simulink model "inversor"  (R2017a)
settings: Solver=FixedStepAuto  StartTime=0.0  StopTime=10.0  FixedStep=1/60/10000  RelTol=1e-3
undefined symbols (not defined in the file): C1, L1, La, R1
libraries: powerlib x15, powerlib_extras x1, simulink x1
settings Model: Creator=Administrador  LastModifiedBy=Administrador
settings OptimizationCC: DefaultParameterBehavior=Inlined  PassReuseOutputArgsAs=Individual arguments
settings DebuggingCC: ParameterTunabilityLossMsg=error
settings SFSimCC: MATLABDynamicMemAlloc=off
settings RTWCC: SystemTargetFile=ert.tlc  TemplateMakefile=ert_default_tmf  Description=Embedded Coder  GenerateReport=on  IncludeHyperlinkInReport=on  LaunchReport=on  GenerateTraceInfo=on  GenerateTraceReport=on  GenerateTraceReportSl=on  GenerateTraceReportSf=on  GenerateTraceReportEml=on
settings CodeAppCC: ForceParamTrailComments=on  IgnoreCustomStorageClasses=off  OperatorAnnotations=on  SimulinkDataObjDesc=on  SFDataObjDesc=on  MATLABFcnDesc=on  InsertBlockDesc=on  MATLABSourceComments=on
settings ERTTargetCC: TargetLangStandard=C99 (ISO)  GenerateSampleERTMain=on  SupportContinuousTime=on  InlinedParameterPlacement=NonHierarchical  ERTCustomFileTemplate=example_file_process.tlc

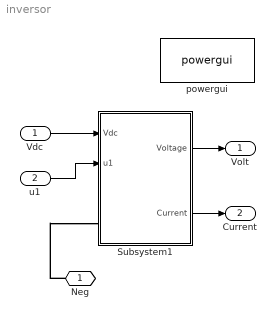
== system inversor ==
  Vdc : Inport
  u1 : Inport  Port=2
  Subsystem1 : Subsystem
  powergui : powerlib/powergui  SimulationMode=Discrete  SampleTime=1/60/10000  frequency=60  Iterations=50  frequencyindice=0  Pbase=100e6  ErrMax=1e-4  UnitsV=kV  UnitsW=MW  buscounter=0  FunctionMessages=off  echomessages=off  EnableUseOfTLC=off  CurrentSourceSwitches=off  DisableSnubberDevices=off  DisableRonSwitches=off  DisableVfSwitches=off  DisplayEquations=off  SolverType=Tustin/Backward Euler (TBE)  Interpol=off  ExternalGateDelay=off  methode=off  Ts=100  x0status=blocks  SPID=off  SwTol=0  HookPort=off  RestoreLinks=warning  ResistiveCurrentMeasurement=off  Frange=[0:2:500]  Ylog=off  Xlog=on  ShowGrid=off  save=off  variable=ZData  structure=sps1phPWM1_str  ZoomFFT=on  StartTime=0.1-2/60  cycles=2  DisplayStyle=1  fundamental=60  FreqAxis=off  MaxFrequency=5000  frequencyindicesteady=1  RmsSteady=1  display=off
  Neg : PMIOPort  Port=1  Side=Left
  Volt : Outport
  Current : Outport  Port=2
  wires:
  Vdc/1 -> Subsystem1/1(Vdc)
  u1/1 -> Subsystem1/2(u1)
  Subsystem1/1(Voltage) -> Volt/1
  Subsystem1/2(Current) -> Current/1
  connections:
  Neg/RConn1 -- Subsystem1/LConn2

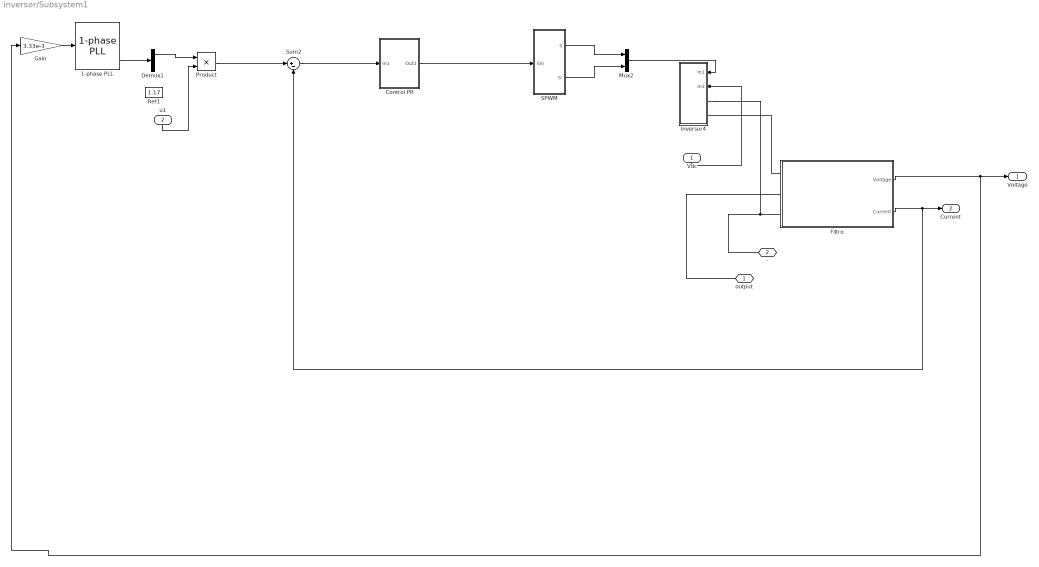
== system inversor/Subsystem1 ==
  Vdc : Inport
  u1 : Inport  Port=2
  1-phase PLL : powerlib_extras/Control  Blocks/1-phase PLL  Par_Init=[0 60]  ParK=[ 180 3200 1 ]  AGC=off
  Control PR : Subsystem
  Demux1 : Demux  Outputs=2
  Filtro : Subsystem
  Gain : Gain  Gain=3.33e-3
  Inversor4 : Subsystem
  Mux2 : Mux  Inputs=2
  Product : Product
  Ref1 : Constant  Value=1.17
  SPWM : Subsystem
  Sum2 : Sum  Inputs=|+-
  output : PMIOPort  Port=1  Side=Left
  - : PMIOPort  Port=2  Side=Left
  Voltage : Outport
  Current : Outport  Port=2
  wires:
  Filtro/2(Current) -> Sum2/2, Current/1
  Filtro/1(Voltage) -> Gain/1, Voltage/1
  1-phase PLL/3 -> Demux1/1
  Gain/1 -> 1-phase PLL/1
  Product/1 -> Sum2/1
  Demux1/1 -> Product/1
  SPWM/1(S) -> Mux2/1
  SPWM/2(S') -> Mux2/2
  Mux2/1 -> Inversor4/1(In1)
  Vdc/1 -> Inversor4/2(In3)
  Control PR/1(Out1) -> SPWM/1(Sin)
  Sum2/1 -> Control PR/1(In1)
  u1/1 -> Product/2
  connections:
  output/RConn1 -- Filtro/LConn2
  -/RConn1 -- Inversor4/LConn1 -- Filtro/LConn3
  Filtro/LConn1 -- Inversor4/LConn2

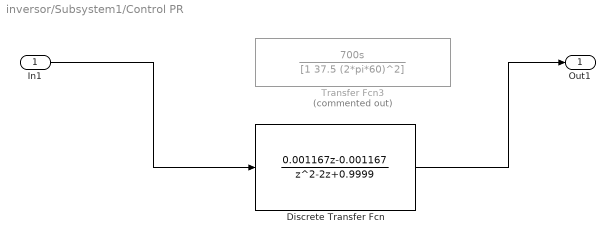
== system inversor/Subsystem1/Control PR ==
  In1 : Inport
  Discrete Transfer Fcn : DiscreteTransferFcn  Numerator=[0.001167 -0.001167]  Denominator=[1 -2 0.9999]  SampleTime=1/60/10000
  Transfer Fcn3 : TransferFcn  Commented=on  Numerator=[700 0]  Denominator=[1 37.5 (2*pi*60)^2]
  Out1 : Outport
  wires:
  Discrete Transfer Fcn/1 -> Out1/1
  In1/1 -> Discrete Transfer Fcn/1

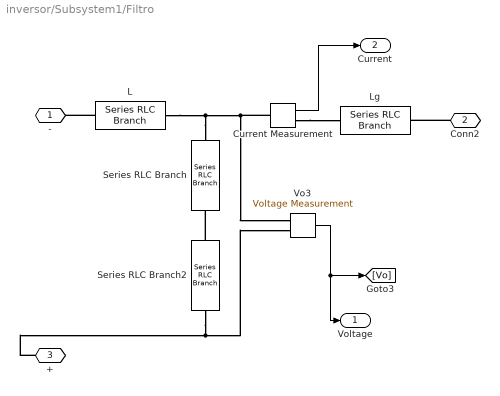
== system inversor/Subsystem1/Filtro ==
  Current Measurement : powerlib/Measurements/Current Measurement  PhasorSimulation=off  OutputType=Complex  PSBequivalent=0
  L : powerlib/Elements/Series RLC Branch  LConnTagsString=__new0  RConnTagsString=__new0  BranchType=RL  Resistance=0.01  Inductance=La  SetiL0=off  InitialCurrent=0  Capacitance=1e-6  Setx0=off  InitialVoltage=0  Measurements=None
  Lg : powerlib/Elements/Series RLC Branch  LConnTagsString=__new0  RConnTagsString=__new0  BranchType=RL  Resistance=R1  Inductance=L1  SetiL0=off  InitialCurrent=0  Capacitance=1e-6  Setx0=off  InitialVoltage=0  Measurements=None
  Series RLC Branch : powerlib/Elements/Series RLC Branch  LConnTagsString=__new0  RConnTagsString=__new0  BranchType=C  Resistance=10  Inductance=25e-3  SetiL0=off  InitialCurrent=0  Capacitance=C1  Setx0=on  InitialVoltage=0  Measurements=None
  Series RLC Branch2 : powerlib/Elements/Series RLC Branch  LConnTagsString=__new0  RConnTagsString=__new0  BranchType=R  Resistance=0.1  Inductance=25e-3  SetiL0=off  InitialCurrent=0  Capacitance=5.30e-3  Setx0=off  InitialVoltage=0  Measurements=None
  Vo3 : powerlib/Measurements/Voltage Measurement  PhasorSimulation=off  OutputType=Complex  PSBequivalent=0
  - : PMIOPort  Port=1  Side=Left
  Conn2 : PMIOPort  Port=2  Side=Left
  + : PMIOPort  Port=3  Side=Left
  Voltage : Outport
  Current : Outport  Port=2
  wires:
  Vo3/1 -> Voltage/1, [Vo]
  Current Measurement/1 -> Current/1
  connections:
  L/LConn1 -- -/RConn1
  Series RLC Branch/LConn1 -- Current Measurement/LConn1 -- Vo3/LConn1 -- L/RConn1
  Series RLC Branch2/LConn1 -- Series RLC Branch/RConn1
  Current Measurement/RConn1 -- Lg/LConn1
  Series RLC Branch2/RConn1 -- +/RConn1 -- Vo3/LConn2
  Conn2/RConn1 -- Lg/RConn1

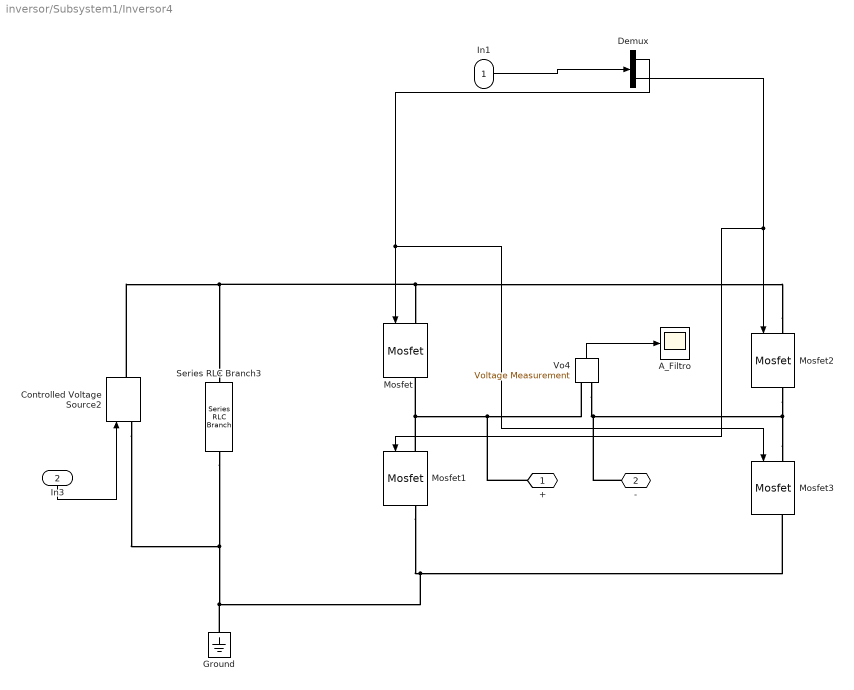
== system inversor/Subsystem1/Inversor4 ==
  In1 : Inport
  In3 : Inport  Port=2
  A_Filtro : Scope
  Controlled Voltage Source2 : powerlib/Electrical Sources/Controlled Voltage Source  Initialize=on  Source_Type=DC  Amplitude=0  Phase=0  Frequency=0  Measurements=None
  Demux : Demux  Outputs=2
  Ground : powerlib/Elements/Ground  LConnTagsString=a
  Mosfet{,1..3} (4 alike) : powerlib/Power Electronics/Mosfet  Ron=0.1  Lon=0  Rd=0.01  Vfd=0  IC=0  Rs=1e5  Cs=inf  Measurements=on
  Series RLC Branch3 : powerlib/Elements/Series RLC Branch  LConnTagsString=__new0  RConnTagsString=__new0  BranchType=RC  Resistance=1  Inductance=25e-3  SetiL0=off  InitialCurrent=0  Capacitance=2.2e-3  Setx0=off  InitialVoltage=0  Measurements=None
  Vo4 : powerlib/Measurements/Voltage Measurement  PhasorSimulation=off  OutputType=Complex  PSBequivalent=0
  + : PMIOPort  Port=1  Side=Left
  - : PMIOPort  Port=2  Side=Left
  wires:
  Vo4/1 -> A_Filtro/1
  Demux/1 -> Mosfet3/1, Mosfet/1
  Demux/2 -> Mosfet1/1, Mosfet2/1
  In3/1 -> Controlled Voltage Source2/1
  In1/1 -> Demux/1
  connections:
  Mosfet3/LConn1 -- -/RConn1 -- Vo4/LConn2 -- Mosfet2/RConn1
  Mosfet2/LConn1 -- Mosfet/LConn1 -- Controlled Voltage Source2/RConn1 -- Series RLC Branch3/LConn1
  Mosfet/RConn1 -- Mosfet1/LConn1 -- Vo4/LConn1 -- +/RConn1
  Mosfet1/RConn1 -- Series RLC Branch3/RConn1 -- Controlled Voltage Source2/LConn1 -- Ground/LConn1 -- Mosfet3/RConn1

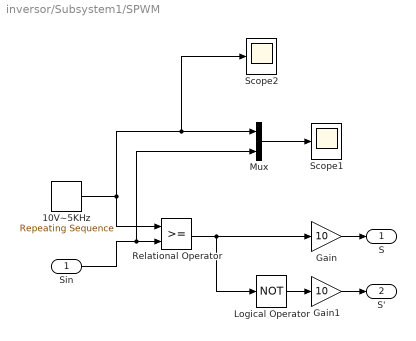
== system inversor/Subsystem1/SPWM ==
  Sin : Inport
  10V~5KHz : simulink/Sources/Repeating Sequence  rep_seq_t=[0 0.0001 0.0002]  rep_seq_y=[-10.5 10.5 -10.5]
  Gain : Gain  Gain=10
  Gain1 : Gain  Gain=10
  Logical Operator : Logic  Operator=NOT  AllPortsSameDT=off  OutDataTypeStr=boolean
  Mux : Mux  Inputs=2
  Relational Operator : RelationalOperator  OutDataTypeStr=boolean  RndMeth=Nearest
  Scope1 : Scope
  Scope2 : Scope
  S : Outport
  S' : Outport  Port=2
  wires:
  10V~5KHz/1 -> Relational Operator/1, Mux/1, Scope2/1
  Relational Operator/1 -> Gain/1, Logical Operator/1
  Logical Operator/1 -> Gain1/1
  Gain/1 -> S/1
  Gain1/1 -> S'/1
  Mux/1 -> Scope1/1
  Sin/1 -> Relational Operator/2, Mux/2
